simulink model "Eocycle_EOX_M26"  (R2022a)
settings: Solver=FixedStepDiscrete  StartTime=0.0  StopTime=50  FixedStep=20e-6  RelTol=1e-7
InitFcn:
  | run('Initialize.m')
values from neighbouring files (symbols this model uses):
  breakpoints = cp_data(2:end,1)'    [Initialize.m]
  C3p = 55e-6    (= 5.5e-05)    [Initialize.m]
  Cdc = 0.1    [Initialize.m]
  dbf = 0.02    [Initialize.m]
  dbV = 0.02    [Initialize.m]
  fnom = 60    [Initialize.m]
  kf = 0.05    [Initialize.m]
  kV = 0.06/0.44    (= 0.136363636364)    [Initialize.m]
  Ldc = 0.06    [Initialize.m]
  Mp = 0.5*rho*pi*rotor_radius^2    (= 325.194109555)    [Initialize.m]
  Power_est = Vdc_data(2:end,3)'    [Initialize.m]
  Prated = 92450    [Initialize.m]
  Qrated = 110000    [Initialize.m]
  R3p = 0.001    [Initialize.m]
  Rdc = 0.001    [Initialize.m]
  rotor_radius = 13    [Initialize.m]
  Ts = 20e-6    (= 2e-05)    [Initialize.m]
  TSR_Cp_table = cp_data(2:end,2)    [Initialize.m]
  Ucutin = 2.75    [Initialize.m]
  Ucutout = 20    [Initialize.m]
  Vdc_nom = 380    [Initialize.m]
  Vdc_set = Vdc_data(2:end,2)'    [Initialize.m]
  Vnom = 480    [Initialize.m]
  wn = (2*pi*N/60)    (= 5.75958653158)    [Initialize.m]
  WS = Vdc_data(2:end,1)'    [Initialize.m]
undefined symbols (not defined in the file or in its folder): breakpoints2, DiscIntNeverNeededParam, magnitude, turbine
libraries: spsSeriesRLCBranchLib x5, simulink x3, eeGeneralControl x3, spsThreePhaseVIMeasurementLib x2, spsGroundLib x2, spsThreePhaseDynamicLoadLib x1, slpidlib x1, spsControlledVoltageSourceLib x1, spsCurrentMeasurementLib x1, spsThreePhaseSeriesRLCLoadLib x1, spsPLL3phLib x1, spsPermanentMagnetSynchronousMachineLib x1
settings Model: SimulationMode=accelerator  Creator=glopezc  LastModifiedBy=banderso2

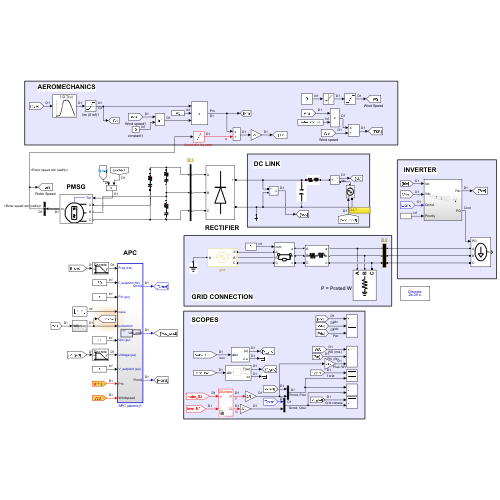
[thumbnail: Simulink's stored preview of the top-level diagram]
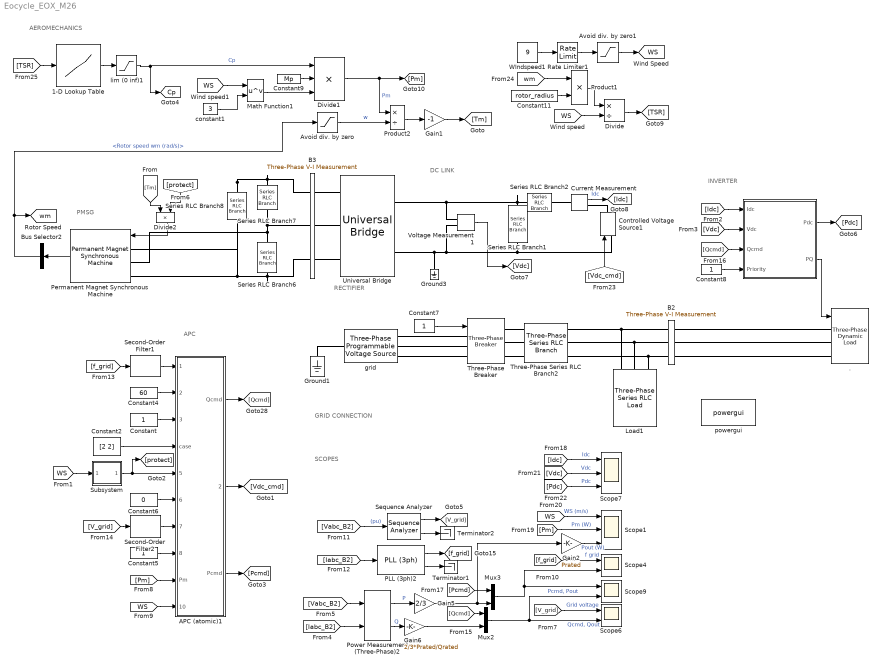
== system Eocycle_EOX_M26 ==
  note: INVERTER
  note: AEROMECHANICS
  note: DC LINK
  note: GRID CONNECTION
  note: SCOPES
  note: APC
  note: PMSG
  note: RECTIFIER
  " " : Subsystem
  . : spsThreePhaseDynamicLoadLib/Three-Phase Dynamic Load  NominalVoltage=[Vnom fnom]  ActiveReactivePowers=[Prated Qrated]  PositiveSequence=[1 0]  ExternalControl=on  NpNq=[1.3 2]  TimeConstants="[0  0  0  0]"  MinimumVoltage=0.7  Tfilter=1e-4  LoadFlowParameters=[4,0,0,0,0]
      settings: SourceProductBaseCode=PS
  1-D Lookup Table : Lookup_n-D  NumberOfTableDimensions=1  BreakpointsForDimension1=breakpoints  BreakpointsForDimension2=turbine.Aero.lambda  Table=TSR_Cp_table  InternalRulePriority=Speed  RndMeth=Simplest
  APC (atomic)1 : Subsystem  TreatAsAtomicUnit=on  SystemSampleTime=2e-5
  "Avoid div. by zero " : Saturate  UpperLimit=inf  LowerLimit=eps
  Avoid div. by zero1 : Saturate  UpperLimit=inf  LowerLimit=eps
  B2 : spsThreePhaseVIMeasurementLib/Three-Phase V-I Measurement  VoltageMeasurement=phase-to-ground  SetLabelV=on  LabelV=Vabc_B2  Vpu=on  VpuLL=off  CurrentMeasurement=yes  SetLabelI=on  LabelI=Iabc_B2  Ipu=on  Pbase=Prated  Vbase=Vnom  OutputType=Magnitude  PhasorSimulation=off  PSBequivalent=0
  B3 : spsThreePhaseVIMeasurementLib/Three-Phase V-I Measurement  VoltageMeasurement=phase-to-ground  SetLabelV=on  LabelV=Vabc_B9  Vpu=off  VpuLL=off  CurrentMeasurement=yes  SetLabelI=on  LabelI=Iabc_B9  Ipu=off  Pbase=100e6  Vbase=440  OutputType=Magnitude  PhasorSimulation=off  PSBequivalent=0
  Bus Selector2 : BusSelector  OutputSignals=Rotor speed wm (rad/s)
  Constant{,5,7..8} (4 alike) : Constant
  Constant11 : Constant  Value=rotor_radius
  Constant2 : Constant  Value=[2 2]
  Constant4 : Constant  Value=60
  Constant6 : Constant  Value=0
  Constant9 : Constant  Value=Mp
  Controlled Voltage Source1 : spsControlledVoltageSourceLib/Controlled Voltage Source  Initialize=on  Source_Type=DC  Amplitude=625  Phase=0  Frequency=60  Measurements=None
  Current Measurement : spsCurrentMeasurementLib/Current Measurement  PhasorSimulation=off  OutputType=Complex  PSBequivalent=0
  Divide : Product  Inputs=*/
  Divide1 : Product  Inputs=***
  Divide2 : Product  Inputs=**
  Gain1 : Gain  Gain=-1
  Gain2 : Gain  Gain=Prated
  Gain5 : Gain  Gain=2/3
  Gain6 : Gain  Gain=2/3*Prated/Qrated
  Ground1 : spsGroundLib/Ground  LConnTagsString=a
  Ground3 : spsGroundLib/Ground  LConnTagsString=a
  Load1 : spsThreePhaseSeriesRLCLoadLib/Three-Phase Series RLC Load  LConnTagsString=A|B|C  Configuration=Y (grounded)  NominalVoltage=Vnom  Vabc=[1e3 1e3 1e3]  Vabcp=[1e3 1e3 1e3]  NominalFrequency=fnom  UnbalancedPower=off  ActivePower=Prated  InductivePower=0  CapacitivePower=0  Pabc=[10e3 9e3 11e3]  QLabc=[100 90 110]  QCabc=[100 90 110]  Pabcp=[10e3 9e3 11e3]  QLabcp=[100 90 110]  QCabcp=[100 90 110]  Measurements=None  LoadType=constant Z
      settings: AttributesFormatString=P = %<ActivePower> W
  Math Function1 : Math  Operator=pow
  Mux2 : Mux  Inputs=2
  Mux3 : Mux  Inputs=2
  PLL (3ph)2 : spsPLL3phLib/PLL (3ph)  Fmin=45  Par_Init=[0, 60]  ParK=[180, 3200, 1]  TcD=1e-4  MaxRateChangeFreq=12  FilterCutOffFreq=25  Ts=Ts  AGC=on
  Permanent Magnet Synchronous Machine : spsPermanentMagnetSynchronousMachineLib/Permanent Magnet Synchronous Machine  NbPhases=3  FluxDistribution=Sinusoidal  RotorType=Round  MechanicalLoad=Torque Tm  PresetModel=No  ShowDetailedParameters=on  MeasurementBus=off  Resistance=0.1  Inductance=8.5e-3  dqInductances=[0.0128 0.0128]  La=0.000164  MachineConstant=Voltage Constant (V_peak L-L / krpm)  Flux=2.3792  VoltageCst=8630.74  TorqueCst=71.3756  Flat=120  Mechanical=[1750 0 20 0]  PolePairs=4  InitialConditions=[wn,0, 0,0]  InitialConditions5ph=[0 0 0 0 0 0]  RefAngle=90 degrees behind phase A axis (modified Park)  IterativeDiscreteModel=Trapezoidal non iterative  TsBlock=-1  TsPowergui=0
  Power Measurement (Three-Phase)2 : eePowerMeasurement/Power Measurement (Three-Phase)  LabelModeActiveChoice=Discrete  F=60  K=[1]  Seq=Positive  Ts=Ts
      settings: SourceProductBaseCode=PS
  Product1 : Product  Inputs=**  InputSameDT=on  SaturateOnIntegerOverflow=on  OutDataTypeStr=Inherit: Same as first input
  Product2 : Product  Inputs=*/  InputSameDT=on  SaturateOnIntegerOverflow=on  OutDataTypeStr=Inherit: Same as first input
  Rate Limiter1 : RateLimiter  RisingSlewLimit=10  FallingSlewLimit=-10  SampleTimeMode=inherited  InitialCondition=9
  Scope1 : Scope  NumInputPorts=3
  Scope4 : Scope  NumInputPorts=2
  Scope6 : Scope  NumInputPorts=2
  Scope7 : Scope  NumInputPorts=3
  Scope9 : Scope  NumInputPorts=2
  Second-Order Filter1 : eeGeneralControl/Second-Order Filter  FilterType=Low-pass  fn=10  Zeta=0.707  Ts=-1  A0=0  Ph0=0  f0=0  b0=0
      settings: SourceProductBaseCode=PS
  Second-Order Filter2 : eeGeneralControl/Second-Order Filter  FilterType=Low-pass  fn=10  Zeta=0.707  Ts=-1  A0=0  Ph0=0  f0=0  b0=0
      settings: SourceProductBaseCode=PS
  Sequence Analyzer : spsSequenceAnalyzerLib/Sequence Analyzer  Freq=60  n=1  seq=Positive  InInit=[1, 0]  Ts=Ts
      settings: SourceProductBaseCode=PS
  Series RLC Branch1 : spsSeriesRLCBranchLib/Series RLC Branch  LConnTagsString=__new0  RConnTagsString=__new0  BranchType=C  Resistance=.00084  Inductance=1e-3  SetiL0=off  InitialCurrent=0  Capacitance=Cdc  Setx0=off  InitialVoltage=0  Measurements=None
  Series RLC Branch2 : spsSeriesRLCBranchLib/Series RLC Branch  LConnTagsString=__new0  RConnTagsString=__new0  BranchType=RL  Resistance=Rdc  Inductance=Ldc  SetiL0=off  InitialCurrent=0  Capacitance=2200e-6  Setx0=off  InitialVoltage=0  Measurements=None
  Series RLC Branch6 : spsSeriesRLCBranchLib/Series RLC Branch  LConnTagsString=__new0  RConnTagsString=__new0  BranchType=RC  Resistance=R3p  Inductance=1e-3  SetiL0=off  InitialCurrent=0  Capacitance=C3p  Setx0=off  InitialVoltage=0  Measurements=None
  Series RLC Branch7 : spsSeriesRLCBranchLib/Series RLC Branch  LConnTagsString=__new0  RConnTagsString=__new0  BranchType=RC  Resistance=R3p  Inductance=1e-3  SetiL0=off  InitialCurrent=0  Capacitance=C3p  Setx0=off  InitialVoltage=0  Measurements=None
  Series RLC Branch8 : spsSeriesRLCBranchLib/Series RLC Branch  LConnTagsString=__new0  RConnTagsString=__new0  BranchType=RC  Resistance=R3p  Inductance=1e-3  SetiL0=off  InitialCurrent=0  Capacitance=C3p  Setx0=off  InitialVoltage=0  Measurements=None
  Subsystem : Subsystem
  Terminator1 : Terminator
  Terminator2 : Terminator
  Three-Phase Series RLC Branch2 : spsThreePhaseSeriesRLCBranchLib/Three-Phase Series RLC Branch  LConnTagsString=A|B|C  RConnTagsString=A|B|C  BranchType=RL  Resistance=1e-5  Inductance=1e-4  Capacitance=1e-6  Measurements=None
  Three-Phase Breaker : spsThreePhaseBreakerLib/Three-Phase Breaker  InitialState=closed  SwitchA=on  SwitchB=on  SwitchC=on  SwitchTimes="[1/60  5/60]"  External=on  BreakerResistance=0.01  SnubberResistance=1e6  SnubberCapacitance=inf  Measurements=None
  Universal Bridge : spsUniversalBridgeLib/Universal Bridge  Arms=3  SnubberResistance=Rs  SnubberCapacitance=Cs  Device=Diodes  Ron=Ron  Lon=0  ForwardVoltages="[  0  0  ]"  ForwardVoltage=Vf  GTOparameters=[ 10e-6 , 20e-6 ]  IGBTparameters=[ 1e-6 , 2e-6 ]  Measurements=Device currents  Measurements_2=None  converterType=Rectifier
  Voltage Measurement1 : spsVoltageMeasurementLib/Voltage Measurement  PhasorSimulation=off  OutputType=Complex  PSBequivalent=0
  WIndspeed1 : Constant  Value=9
  constant1 : Constant  Value=3
  grid : spsThreePhaseProgrammableVoltageSourceLib/Three-Phase Programmable Voltage Source  PositiveSequence=[Vnom 0 fnom]  VariationEntity=None  VariationType=Table of time-amplitude pairs  VariationTypeAlt=Step  VariationStep=-0.1  VariationRate=10  VariationMagnitude=0.3  VariationFrequency=2  VariationTiming=[10 20]  VariationPhaseA=off  Amplitudes=[1 1 0.9 0.9 1.1 1.1 1 1]  TimeValues=[0 5 5.1 10 10.1 15 15.1 20]  HarmonicGeneration=off  HarmonicA=[1 -0.1 0 2]  HarmonicB=[2 0.15 35 2]*0  Timing="[0.1  2]"  BusType=swing  Pref=0  Qref=0  Qmin=-inf  Qmax=inf
  lim (0 inf)1 : Saturate  UpperLimit=inf  LowerLimit=eps
  powergui : spspowerguiLib/powergui  Priority=1  SimulationMode=Discrete  SampleTime=20e-6  frequency=60  Iterations=50  frequencyindice=0  Pbase=100e6  ErrMax=1e-4  UnitsV=kV  UnitsW=MW  buscounter=0  FunctionMessages=off  echomessages=off  EnableUseOfTLC=off  CurrentSourceSwitches=off  DisableSnubberDevices=off  DisableRonSwitches=off  DisableVfSwitches=off  DisplayEquations=off  AutomaticDiscreteSolvers=off  SolverType=Tustin/Backward Euler (TBE)  Interpol=off  ExternalGateDelay=off  methode=off  Ts=100  x0status=blocks  SPID=on  SwTol=0  HookPort=off  NonlinearTolerance=1e-7  nMaxIteration=150  ContinueOnMaxIteration=off  RestoreLinks=warning  ResistiveCurrentMeasurement=off  Frange=[0:2:500]  Ylog=off  Xlog=on  ShowGrid=off  save=off  variable=ZData  structure=0  ZoomFFT=off  StartTime=0.0  cycles=1  DisplayStyle=1  fundamental=60  FreqAxis=off  MaxFrequency=1000  frequencyindicesteady=1  RmsSteady=1  display=off
  tag scope: Cp=global, WS=global, wm=global
  wires:
  [Vabc_B2] -> Power Measurement (Three-Phase)2/1
  [Iabc_B2] -> Power Measurement (Three-Phase)2/2
  Power Measurement (Three-Phase)2/2 -> Gain6/1  "Q"
  Power Measurement (Three-Phase)2/1 -> Gain5/1  "P"
  [Vabc_B2] -> Sequence Analyzer/1  "(pu)"
  Sequence Analyzer/1 -> [V_grid]
  [Iabc_B2] -> PLL (3ph)2/1
  PLL (3ph)2/1 -> [f_grid]
  PLL (3ph)2/2 -> Terminator1/1
  Second-Order Filter1/1 -> APC (atomic)1/1(Freq (Hz))
  Constant2/1 -> APC (atomic)1/4(case)
  Constant4/1 -> APC (atomic)1/2(f_setpoint (Hz))
  APC (atomic)1/1(Qcmd) -> [Qcmd]
  Constant6/1 -> APC (atomic)1/6(Qin (pu))
  Constant/1 -> APC (atomic)1/3(Pin (pu))
  Constant5/1 -> APC (atomic)1/8(V_setpoint (pu))
  Sequence Analyzer/2 -> Terminator2/1
  APC (atomic)1/2(Vdc_cmd) -> [Vdc_cmd]
  [Pm] -> APC (atomic)1/9(Pm)
  [WS] -> APC (atomic)1/10(Windspeed)
  [f_grid] -> Scope4/1  "f grid"
  [Qcmd] -> Mux2/1
  Mux2/1 -> Scope9/2, Scope6/2  "Qcmd, Qout"
  APC (atomic)1/3(Pcmd) -> [Pcmd]
  [Pcmd] -> Mux3/1
  Mux3/1 -> Scope9/1, Scope4/2  "Pcmd, Pout"
  [V_grid] -> Scope6/1  "Grid voltage"
  Gain5/1 -> Gain2/1, Mux3/2
  Gain6/1 -> Mux2/2
  [f_grid] -> Second-Order Filter1/1
  [V_grid] -> Second-Order Filter2/1
  Second-Order Filter2/1 -> APC (atomic)1/7(Voltage (pu))
  Current Measurement/1 -> [Idc]  "Idc"
  Constant7/1 -> Three-Phase Breaker/1
  [Pm] -> Scope1/2  "Pm (W)"
  [WS] -> Scope1/1  "WS (m/s)"
  [Idc] -> Scope7/1  "Idc"
  [Vdc] -> Scope7/2  "Vdc"
  [Pdc] -> Scope7/3  "Pdc"
  [Idc] -> " "/1(Idc)
  [Vdc] -> " "/2(Vdc)
  Constant8/1 -> " "/4(Priority)
  [Qcmd] -> " "/3(Qcmd)
  " "/1(Pdc) -> [Pdc]
  " "/2(PQ) -> ./1
  Gain2/1 -> Scope1/3  "Pout (W)"
  Rate Limiter1/1 -> Avoid div. by zero1/1
  [wm] -> Product1/1
  WIndspeed1/1 -> Rate Limiter1/1
  Divide/1 -> [TSR]
  Avoid div. by zero1/1 -> [WS]
  Product1/1 -> Divide/1
  [WS] -> Divide/2
  Gain1/1 -> [Tm]
  [WS] -> Math Function1/1
  constant1/1 -> Math Function1/2
  "Avoid div. by zero "/1 -> Product2/2  "w"
  Math Function1/1 -> Divide1/3
  Product2/1 -> Gain1/1
  lim (0 inf)1/1 -> [Cp], Divide1/1  "Cp"
  Constant9/1 -> Divide1/2
  Divide1/1 -> [Pm], Product2/1  "Pm"
  Bus Selector2/1 -> "Avoid div. by zero "/1, [wm]  "<Rotor speed wm (rad/s)>"
  Permanent Magnet Synchronous Machine/1 -> Bus Selector2/1
  Divide2/1 -> Permanent Magnet Synchronous Machine/1
  Voltage Measurement1/1 -> [Vdc]
  [TSR] -> 1-D Lookup Table/1
  1-D Lookup Table/1 -> lim (0 inf)1/1
  [Vdc_cmd] -> Controlled Voltage Source1/1
  Constant11/1 -> Product1/2
  Subsystem/1(Protection) -> APC (atomic)1/5(protection), [protect]
  [WS] -> Subsystem/1(WS)
  [Tm] -> Divide2/1
  [protect] -> Divide2/2
  connections:
  Voltage Measurement1/LConn2 -- Series RLC Branch1/RConn1 -- Controlled Voltage Source1/LConn1 -- Ground3/LConn1 -- Universal Bridge/RConn2
  B2/RConn1 -- Three-Phase Series RLC Branch2/RConn1 -- Load1/LConn1
  Load1/LConn3 -- B2/RConn3 -- Three-Phase Series RLC Branch2/RConn3
  Load1/LConn2 -- Three-Phase Series RLC Branch2/RConn2 -- B2/RConn2
  Three-Phase Breaker/LConn3 -- grid/RConn3
  Three-Phase Breaker/LConn2 -- grid/RConn2
  Three-Phase Breaker/LConn1 -- grid/RConn1
  B2/LConn1 -- ./LConn1
  B2/LConn2 -- ./LConn2
  B2/LConn3 -- ./LConn3
  Ground1/LConn1 -- grid/LConn1
  Current Measurement/RConn1 -- Controlled Voltage Source1/RConn1
  Series RLC Branch1/LConn1 -- Universal Bridge/RConn1 -- Voltage Measurement1/LConn1 -- Series RLC Branch2/LConn1
  Three-Phase Breaker/RConn1 -- Three-Phase Series RLC Branch2/LConn1
  Three-Phase Breaker/RConn2 -- Three-Phase Series RLC Branch2/LConn2
  Three-Phase Breaker/RConn3 -- Three-Phase Series RLC Branch2/LConn3
  Current Measurement/LConn1 -- Series RLC Branch2/RConn1
  Series RLC Branch6/LConn1 -- Series RLC Branch7/RConn1 -- B3/RConn2 -- Permanent Magnet Synchronous Machine/LConn2
  Series RLC Branch8/RConn1 -- Series RLC Branch6/RConn1 -- B3/RConn3 -- Permanent Magnet Synchronous Machine/LConn3
  Permanent Magnet Synchronous Machine/LConn1 -- Series RLC Branch7/LConn1 -- B3/RConn1 -- Series RLC Branch8/LConn1
  B3/LConn2 -- Universal Bridge/LConn2
  B3/LConn3 -- Universal Bridge/LConn3
  B3/LConn1 -- Universal Bridge/LConn1

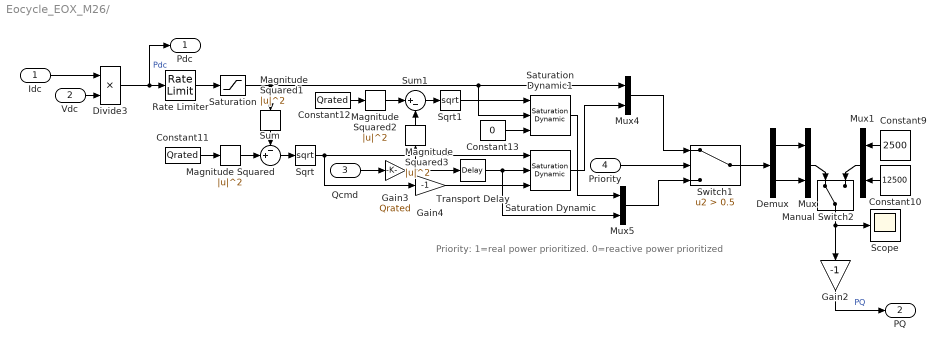
== system Eocycle_EOX_M26/  ==
  note: Priority: 1=real power prioritized. 0=reactive power prioritized
  Idc : Inport
  Vdc : Inport  Port=2
  Qcmd : Inport  Port=3
  Priority : Inport  Port=4
  Constant10 : Constant  Value=12500
  Constant11 : Constant  Value=Qrated
  Constant12 : Constant  Value=Qrated
  Constant13 : Constant  Value=0
  Constant9 : Constant  Value=2500
  Demux : Demux  Outputs=2
  Divide3 : Product  Inputs=**
  Gain2 : Gain  Gain=-1
  Gain3 : Gain  Gain=Qrated
  Gain4 : Gain  Gain=-1
  Magnitude Squared{,1..3} (4 alike) : Math  Operator=magnitude^2
  Manual Switch2 : ManualSwitch
  Mux{,1,4..5} (4 alike) : Mux  Inputs=2
  Rate Limiter : RateLimiter  RisingSlewLimit=5000  FallingSlewLimit=-5000  SampleTimeMode=inherited  InitialCondition=Prated
  Saturation : Saturate  UpperLimit=Prated*1.1  LowerLimit=0
  Saturation Dynamic : simulink/Discontinuities/Saturation Dynamic  OutMin=[]  OutMax=[]  OutDataTypeStr=Inherit: Same as second input  OutDataType=fixdt(1, 16)  OutScaling=2^-10  DoSatur=off
  Saturation Dynamic1 : simulink/Discontinuities/Saturation Dynamic  OutMin=[]  OutMax=[]  OutDataTypeStr=Inherit: Same as second input  OutDataType=fixdt(1, 16)  OutScaling=2^-10  DoSatur=off
  Scope : Scope
  Sqrt : Sqrt
  Sqrt1 : Sqrt
  Sum : Sum  Inputs=-+|
  Sum1 : Sum  Inputs=|+-
  Switch1 : Switch  Criteria=u2 > Threshold  Threshold=0.5  SaturateOnIntegerOverflow=off  InputSameDT=off
  Transport Delay : TransportDelay  DelayTime=10e-3
  Pdc : Outport
  PQ : Outport  Port=2
  wires:
  Constant13/1 -> Saturation Dynamic1/3
  Magnitude Squared/1 -> Sum/2
  Mux/1 -> Manual Switch2/1
  Manual Switch2/1 -> Scope/1, Gain2/1
  Priority/1 -> Switch1/2
  Constant10/1 -> Mux1/2
  Constant9/1 -> Mux1/1
  Gain4/1 -> Saturation Dynamic/3
  Saturation Dynamic/1 -> Mux4/2
  Transport Delay/1 -> Mux5/2, Saturation Dynamic/2
  Mux1/1 -> Manual Switch2/2
  Sum1/1 -> Sqrt1/1
  Divide3/1 -> Rate Limiter/1, Pdc/1  "Pdc"
  Constant12/1 -> Magnitude Squared2/1
  Qcmd/1 -> Gain3/1
  Constant11/1 -> Magnitude Squared/1
  Sqrt/1 -> Gain4/1, Saturation Dynamic/1
  Mux4/1 -> Switch1/1
  Magnitude Squared1/1 -> Sum/1
  Sum/1 -> Sqrt/1
  Magnitude Squared2/1 -> Sum1/1
  Mux5/1 -> Switch1/3
  Gain3/1 -> Transport Delay/1, Magnitude Squared3/1
  Saturation Dynamic1/1 -> Mux5/1
  Switch1/1 -> Demux/1
  Vdc/1 -> Divide3/2
  Sqrt1/1 -> Saturation Dynamic1/1
  Idc/1 -> Divide3/1
  Magnitude Squared3/1 -> Sum1/2
  Demux/2 -> Mux/2
  Demux/1 -> Mux/1
  Gain2/1 -> PQ/1  "PQ"
  Saturation/1 -> Saturation Dynamic1/2, Mux4/1, Magnitude Squared1/1
  Rate Limiter/1 -> Saturation/1

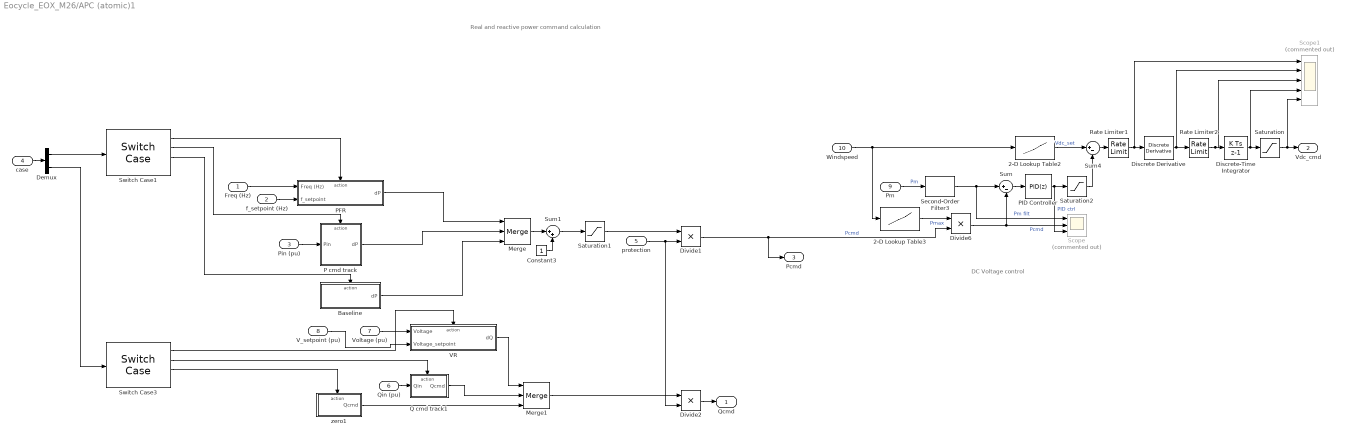
== system Eocycle_EOX_M26/APC (atomic)1 ==
  note: Real and reactive power command calculation
  note: DC Voltage control
  Freq (Hz) : Inport
  f_setpoint (Hz) : Inport  Port=2
  Pin (pu) : Inport  Port=3
  case : Inport  Port=4
  protection : Inport  Port=5
  Qin (pu) : Inport  Port=6
  Voltage (pu) : Inport  Port=7
  V_setpoint (pu) : Inport  Port=8
  Pm : Inport  Port=9
  Windspeed : Inport  Port=10
  2-D Lookup Table2 : Lookup_n-D  NumberOfTableDimensions=1  BreakpointsForDimension1=WS  BreakpointsForDimension2=breakpoints2  BreakpointsForDimension1DataTypeStr=double  BreakpointsForDimension2DataTypeStr=double  Table=Vdc_set  InternalRulePriority=Speed  OutDataTypeStr=double  RndMeth=Simplest
  2-D Lookup Table3 : Lookup_n-D  NumberOfTableDimensions=1  BreakpointsForDimension1=WS  BreakpointsForDimension2=breakpoints2  BreakpointsForDimension1DataTypeStr=double  BreakpointsForDimension2DataTypeStr=double  Table=Power_est  InternalRulePriority=Speed  OutDataTypeStr=double  RndMeth=Simplest
  Baseline : Subsystem
  Constant3 : Constant
  Demux : Demux  Outputs=2
  Discrete Derivative : simulink/Discrete/Discrete Derivative  gainval=1.0  ICPrevScaledInput=0  OutMin=[]  OutMax=[]  OutDataType=fixdt(1, 16)  OutScaling=2^-10  DoSatur=off
  Discrete-Time Integrator : DiscreteIntegrator  InitialCondition=Vdc_nom  SampleTime=-1  ICPrevOutput=DiscIntNeverNeededParam  ICPrevScaledInput=DiscIntNeverNeededParam
  Divide1 : Product  Inputs=**
  Divide2 : Product  Inputs=**
  Divide6 : Product  Inputs=**
  Merge : Merge  Inputs=3
  Merge1 : Merge  Inputs=3
  P cmd track : Subsystem
  PFR : Subsystem
  PID Controller : slpidlib/PID Controller  Controller=PID  Form=Parallel  TimeDomain=Discrete-time  UseExternalTs=off  SampleTime=-1  IntegratorMethod=Forward Euler  FilterMethod=Forward Euler  ControllerParametersSource=internal  P=Vdc_nom/Prated*2.9  I=0  UseKiTs=off  D=0  N=100  UseFilter=on  TunerSelectOption=Transfer Function Based (PID Tuner App)  InitialConditionSource=internal  InitialConditionForIntegrator=0  InitialConditionForFilter=0  DifferentiatorICPrevScaledInput=0  ExternalReset=none  TrackingMode=off  Kt=1  LimitOutput=on  SatLimitsSource=internal  UpperSaturationLimit=inf  LowerSaturationLimit=-inf  LinearizeAsGain=on  AntiWindupMode=back-calculation  Kb=1  POutMin=[]  POutMax=[]  IOutMin=[]  IOutMax=[]  DOutMin=[]  DOutMax=[]  NOutMin=[]  NOutMax=[]  SumOutMin=[]  SumOutMax=[]  SaturationOutMin=[]  SaturationOutMax=[]  PParamMin=[]  PParamMax=[]  IParamMin=[]  IParamMax=[]  DParamMin=[]  DParamMax=[]  NParamMin=[]  NParamMax=[]  KbParamMin=[]  KbParamMax=[]  KtParamMin=[]  KtParamMax=[]  KbOutMin=[]  KbOutMax=[]  KtOutMin=[]  KtOutMax=[]  IntegratorOutMin=[]  IntegratorOutMax=[]  FilterOutMin=[]  FilterOutMax=[]  SumI1OutMin=[]  SumI1OutMax=[]  SumI2OutMin=[]  SumI2OutMax=[]  SumI3OutMin=[]  SumI3OutMax=[]  SumI4OutMin=[]  SumI4OutMax=[]  SumDOutMin=[]  SumDOutMax=[]  DifferentiatorOutMin=[]  DifferentiatorOutMax=[]  FilterDiffOutCoefMin=[]  FilterDiffOutCoefMax=[]  ReciprocalOutMin=[]  ReciprocalOutMax=[]  SumDenOutMin=[]  SumDenOutMax=[]  SumNumOutMin=[]  SumNumOutMax=[]  DivideOutMin=[]  DivideOutMax=[]  UdiffTsProdOutMin=[]  UdiffTsProdOutMax=[]  NTsProdOutMin=[]  NTsProdOutMax=[]  UintegralTsProdOutMin=[]  UintegralTsProdOutMax=[]  UngainTsProdOutMin=[]  UngainTsProdOutMax=[]  IntegratorContinuousStateAttributes=''  IntegratorStateMustResolveToSignalObject=off  IntegratorRTWStateStorageClass=Auto  FilterContinuousStateAttributes=''  FilterStateMustResolveToSignalObject=off  FilterRTWStateStorageClass=Auto  ParallelPVariant=InternalParameters  IdealPVariant=Disabled  IVariant=InternalParameters  DVariant=InternalParameters  IntegratorVariant=Discrete  SatVariant=Enabled  AWVariant=BackCalculation  PCopyVariant=Disabled  TRVariant=Disabled  FdbkBlocksVariant=Forward  IdealPFdbkVariant=Disabled  SatFdbkVariant=Disabled  DerivativeFilterVariant=ForwardEulerFilter  NVariant=InternalParameters  NCopyVariant=Disabled  FilterICVariant=InternalICsFilter  IntegratorICVariant=InternalICs  ExternalResetVariant=Disabled  TRSumVariant=Passthrough  SumFdbkVariant=Disabled  SumVariant=Sum_PID  TsampFilterVariant=InternalTs  TsampNgainVariant=Passthrough  TsampIntegralVariant=Passthrough  ExternalSaturationOutDataTypeStr=Inherit: Same as second input  aMode=0
  Q cmd track1 : Subsystem
  Rate Limiter1 : RateLimiter  RisingSlewLimit=50  FallingSlewLimit=-50  SampleTimeMode=inherited  InitialCondition=Vdc_nom
  Rate Limiter2 : RateLimiter  RisingSlewLimit=500  FallingSlewLimit=-500  SampleTimeMode=inherited
  Saturation : Saturate  UpperLimit=2000  LowerLimit=100
  Saturation1 : Saturate  UpperLimit=1.2  LowerLimit=0.2
  Saturation2 : Saturate  UpperLimit=inf  LowerLimit=0
  Scope : Scope  Commented=on  NumInputPorts=3
  Scope1 : Scope  Commented=on  NumInputPorts=5
  Second-Order Filter3 : eeGeneralControl/Second-Order Filter  FilterType=Low-pass  fn=10  Zeta=0.707  Ts=-1  A0=1150  Ph0=0  f0=0  b0=0
      settings: SourceProductBaseCode=PS
  Sum : Sum  Inputs=|+-
  Sum1 : Sum  Inputs=|++
  Sum4 : Sum  Inputs=|+-
  Switch Case1 : SwitchCase  CaseConditions={1,2,3}
  Switch Case3 : SwitchCase  CaseConditions={1,2,3}
  VR : Subsystem
  zero1 : Subsystem
  Qcmd : Outport
  Vdc_cmd : Outport  Port=2
  Pcmd : Outport  Port=3
  wires:
  Saturation1/1 -> Divide1/1
  Merge1/1 -> Divide2/1
  protection/1 -> Divide2/2, Divide1/2
  Divide2/1 -> Qcmd/1
  P cmd track/1(dP) -> Merge/2
  Constant3/1 -> Sum1/2
  Pin (pu)/1 -> P cmd track/1(Pin)
  PFR/1(dP) -> Merge/1
  Freq (Hz)/1 -> PFR/1(Freq (Hz))
  Merge/1 -> Sum1/1
  Sum1/1 -> Saturation1/1
  Baseline/1(dP) -> Merge/3
  f_setpoint (Hz)/1 -> PFR/2(f_setpoint)
  case/1 -> Demux/1
  Demux/1 -> Switch Case1/1
  Switch Case1/1 -> PFR/Action
  Switch Case1/2 -> P cmd track/Action
  Switch Case1/3 -> Baseline/Action
  Demux/2 -> Switch Case3/1
  Switch Case3/3 -> zero1/Action
  zero1/1(Qcmd) -> Merge1/3
  Switch Case3/2 -> Q cmd track1/Action
  Q cmd track1/1(Qcmd) -> Merge1/2
  Qin (pu)/1 -> Q cmd track1/1(Qin)
  Voltage (pu)/1 -> VR/1("Voltage ")
  V_setpoint (pu)/1 -> VR/2(Voltage_setpoint)
  Switch Case3/1 -> VR/Action
  VR/1(dQ) -> Merge1/1
  2-D Lookup Table3/1 -> Divide6/1  "Pmax"
  2-D Lookup Table2/1 -> Sum4/1  "Vdc_set"
  Pm/1 -> Second-Order Filter3/1  "Pm"
  Divide6/1 -> Sum/2, Scope/2  "Pcmd"
  Sum/1 -> PID Controller/1
  Windspeed/1 -> 2-D Lookup Table3/1, 2-D Lookup Table2/1
  Second-Order Filter3/1 -> Scope/1, Sum/1  "Pm filt"
  Divide1/1 -> Divide6/2, Pcmd/1  "Pcmd"
  Rate Limiter1/1 -> Discrete Derivative/1, Scope1/1
  Discrete Derivative/1 -> Scope1/2, Rate Limiter2/1
  Rate Limiter2/1 -> Scope1/3, Discrete-Time Integrator/1
  Saturation/1 -> Vdc_cmd/1, Scope1/5
  PID Controller/1 -> Scope/3, Saturation2/1  "PID ctrl"
  Discrete-Time Integrator/1 -> Scope1/4, Saturation/1
  Sum4/1 -> Rate Limiter1/1
  Saturation2/1 -> Sum4/2

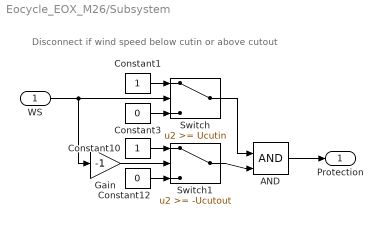
== system Eocycle_EOX_M26/Subsystem ==
  note: Disconnect if wind speed below cutin or above cutout
  WS : Inport
  AND : Logic  IconShape=distinctive  AllPortsSameDT=off  OutDataTypeStr=boolean
  Constant1 : Constant
  Constant10 : Constant
  Constant12 : Constant  Value=0
  Constant3 : Constant  Value=0
  Gain : Gain  Gain=-1
  Switch : Switch  Threshold=Ucutin  SaturateOnIntegerOverflow=off  InputSameDT=off
  Switch1 : Switch  Threshold=-Ucutout  SaturateOnIntegerOverflow=off  InputSameDT=off
  Protection : Outport
  wires:
  Constant3/1 -> Switch/3
  Gain/1 -> Switch1/2
  Constant1/1 -> Switch/1
  Constant12/1 -> Switch1/3
  WS/1 -> Gain/1, Switch/2
  Constant10/1 -> Switch1/1
  Switch/1 -> AND/1
  Switch1/1 -> AND/2
  AND/1 -> Protection/1

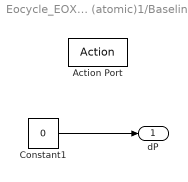
== system Eocycle_EOX_M26/APC (atomic)1/Baseline ==
  Action Port : ActionPort  ActionPortLabel=case [ 3 ]:
  Constant1 : Constant  Value=0
  dP : Outport
  wires:
  Constant1/1 -> dP/1

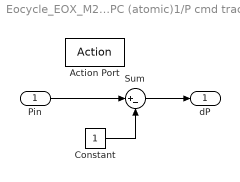
== system Eocycle_EOX_M26/APC (atomic)1/P cmd track ==
  Pin : Inport
  Action Port : ActionPort  ActionPortLabel=case [ 2 ]:
  Constant : Constant
  Sum : Sum  Inputs=|+-
  dP : Outport
  wires:
  Constant/1 -> Sum/2
  Sum/1 -> dP/1
  Pin/1 -> Sum/1

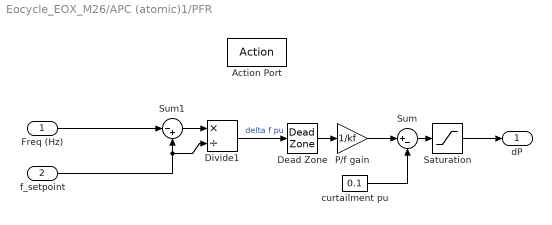
== system Eocycle_EOX_M26/APC (atomic)1/PFR ==
  Freq (Hz) : Inport
  f_setpoint : Inport  Port=2
  Action Port : ActionPort  ActionPortLabel=case [ 1 ]:
  Dead Zone : DeadZone  LowerValue=-dbf/60  UpperValue=dbf/60
  Divide1 : Product  Inputs=*/
  P/f gain : Gain  Gain=1/kf
  Saturation : Saturate  UpperLimit=0  LowerLimit=-0.8
  Sum : Sum  Inputs=|+-
  Sum1 : Sum  Inputs=|-+
  curtailment pu : Constant  Value=0.1
  dP : Outport
  wires:
  Sum/1 -> Saturation/1
  Saturation/1 -> dP/1
  P/f gain/1 -> Sum/1
  curtailment pu/1 -> Sum/2
  Dead Zone/1 -> P/f gain/1
  Freq (Hz)/1 -> Sum1/1
  Divide1/1 -> Dead Zone/1  "delta f pu"
  Sum1/1 -> Divide1/1
  f_setpoint/1 -> Sum1/2, Divide1/2

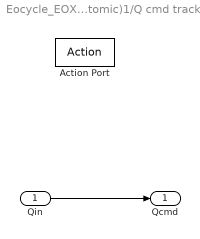
== system Eocycle_EOX_M26/APC (atomic)1/Q cmd track1 ==
  Qin : Inport
  Action Port : ActionPort  ActionPortLabel=case [ 2 ]:
  Qcmd : Outport
  wires:
  Qin/1 -> Qcmd/1

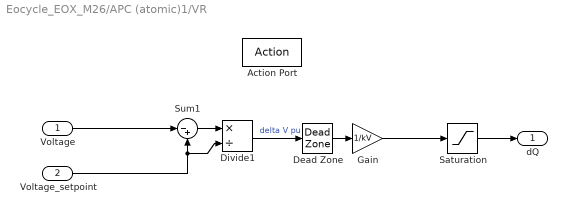
== system Eocycle_EOX_M26/APC (atomic)1/VR ==
  "Voltage " : Inport
  Voltage_setpoint : Inport  Port=2
  Action Port : ActionPort  ActionPortLabel=case [ 1 ]:
  Dead Zone : DeadZone  LowerValue=-dbV  UpperValue=dbV
  Divide1 : Product  Inputs=*/
  Gain : Gain  Gain=1/kV
  Saturation : Saturate  UpperLimit=1  LowerLimit=-1
  Sum1 : Sum  Inputs=|-+
  dQ : Outport
  wires:
  Gain/1 -> Saturation/1
  Saturation/1 -> dQ/1
  Dead Zone/1 -> Gain/1
  "Voltage "/1 -> Sum1/1
  Divide1/1 -> Dead Zone/1  "delta V pu"
  Sum1/1 -> Divide1/1
  Voltage_setpoint/1 -> Divide1/2, Sum1/2

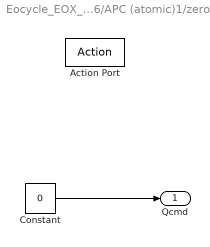
== system Eocycle_EOX_M26/APC (atomic)1/zero1 ==
  Action Port : ActionPort  ActionPortLabel=case [ 3 ]:
  Constant : Constant  Value=0
  Qcmd : Outport
  wires:
  Constant/1 -> Qcmd/1
